simulink model "ElectricVehicle_model_in_the_loop_controller"  (Simulink 8.2)
settings: Solver=ode1  StartTime=0.0  StopTime=42  FixedStep=0.0005  RelTol=1e-3
settings Model: Creator=msdtfa  LastModifiedBy=msdtfa
settings DataIOCC: SignalLoggingName=sigsOut
settings OptimizationCC: ExpressionDepthLimit=128
settings DebuggingCC: SaveWithParameterizedLinksMsg=none  SignalResolutionControl=TryResolveAllWithWarning  SolverPrmCheckMsg=none  MultiTaskDSMMsg=warning  MultiTaskCondExecSysMsg=none  FcnCallInpInsideContextMsg=EnableAllAsError  StateNameClashWarn=none
settings HardwareCC: TargetUnknown=on
settings RTWCC: IncludeERTFirstTime=on

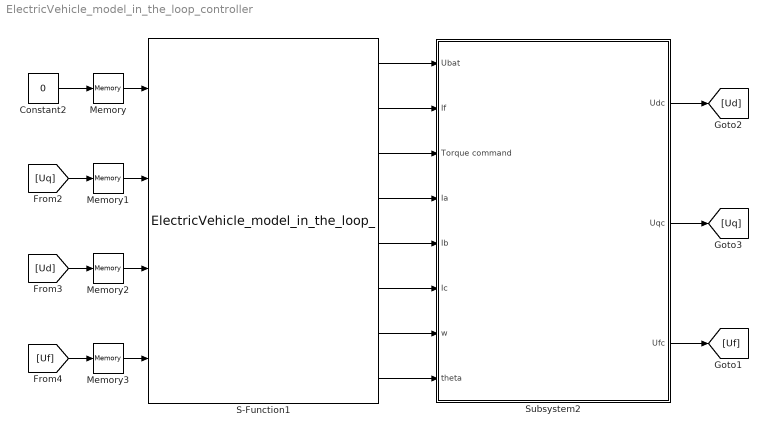
== system ElectricVehicle_model_in_the_loop_controller ==
  Constant2 : Constant  Value=0
  Memory : Memory  InheritSampleTime=on
  Memory1 : Memory  InheritSampleTime=on
  Memory2 : Memory  InheritSampleTime=on
  Memory3 : Memory  X0=500  InheritSampleTime=on
  S-Function1 : S-Function  InitFcn=clear ElectricVehicle_model_in_the_loop_  StopFcn=clear ElectricVehicle_model_in_the_loop_  FunctionName=ElectricVehicle_model_in_the_loop_  Parameters=0.0005 0.01 1e-6  EnableBusSupport=off
      mask Display: port_label('output',1,'Ubat');port_label('output',2,'If');port_label('output',3,'torque_ratio_command');port_label('output',4,'Ia');port_label('output',5,'Ib');port_label('output',6,'Ic');port_label('output',7,'rotary_velocity');port_label('output',8,'mechanical_angle');port_label('input',1,'Uoc');port_label('input',2,'Uqc');port_label('input',3,'Udc');port_label('input',4,'Ufc');disp('Simcenter Amesim:\n ElectricVehicle_model_in_the_loop_')
  Subsystem2 : Subsystem  mask{p=2, Lf=20.8, Rf=35, Tauf=0.01, Msf=0.08, Lsd=0.0006, Lsq=0.0006, Rs=0.08, Taud=0.01, Tauq=0.12, Ifmax=5, Irmsmax=110}
      mask prompts: p "number of pole pairs"; Lf "field winding inductance"; Rf "field winding resistance"; Tauf "field axis PI time constant"; Msf "mutual inductance between stator and field"; Lsd "stator cyclic inductance on Park's d axis"; Lsq "stator cyclic inductance on Park's q axis"; Rs "stator winding resistance"; Taud "d axis PI time constant"; Tauq "q axis PI time constant"; Ifmax "maximum field winding current"; Irmsmax "maximum RMS stator current"
      mask Display:
      | port_label('input',1,'Ubat');
      | port_label('input',2,'If');
      | port_label('input',3,'torque_ratio_c');
      | port_label('input',4,'Ia');
      | port_label('input',5,'Ib');
      | port_label('input',6,'Ic');
      | port_label('input',7,'rotary_velocity');
      | port_label('input',8,'mechanical_angle');
      | port_label('output',1,'Ud');
      | port_label('output',2,'Uq');
      | port_label('output',3,'Uf');
      | 
      | disp('WRSM CONTROL\n Simulink subsystem')
  wires:
  Memory3/1 -> S-Function1/4
  Memory2/1 -> S-Function1/3
  Memory1/1 -> S-Function1/2
  Memory/1 -> S-Function1/1
  Constant2/1 -> Memory/1
  [Uq] -> Memory1/1
  [Uf] -> Memory3/1
  [Ud] -> Memory2/1
  Subsystem2/3(Ufc) -> [Uf]
  Subsystem2/1(Udc) -> [Ud]
  Subsystem2/2(Uqc) -> [Uq]
  S-Function1/3 -> Subsystem2/3(Torque command)
  S-Function1/4 -> Subsystem2/4(Ia)
  S-Function1/5 -> Subsystem2/5(Ib)
  S-Function1/6 -> Subsystem2/6(Ic)
  S-Function1/7 -> Subsystem2/7(w)
  S-Function1/8 -> Subsystem2/8(theta)
  S-Function1/2 -> Subsystem2/2(If)
  S-Function1/1 -> Subsystem2/1(Ubat)

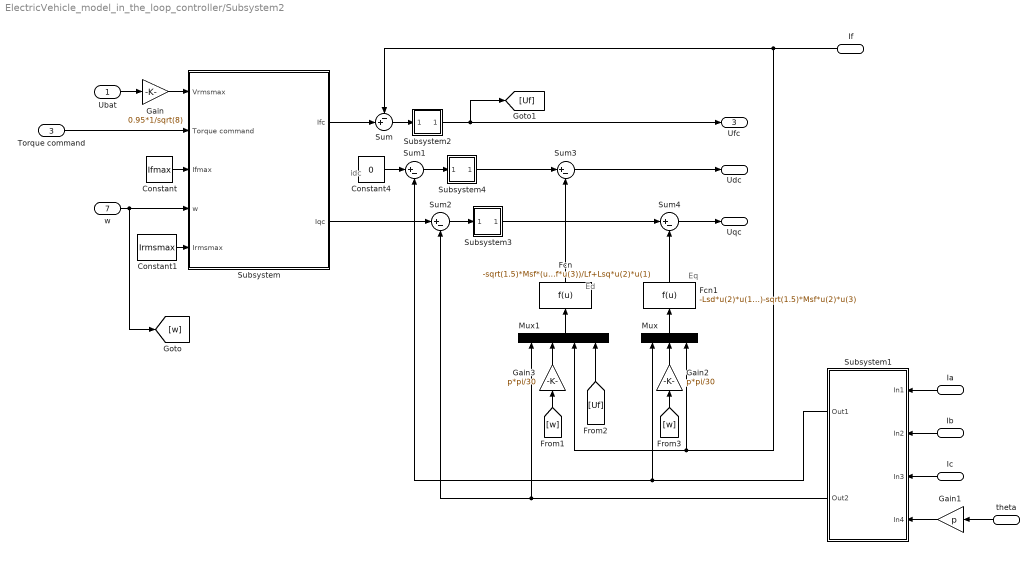
== system ElectricVehicle_model_in_the_loop_controller/Subsystem2 ==
  note: Ed
  note: Eq
  note: idc
  Ubat : Inport
  If : Inport  Port=2
  Torque command : Inport  Port=3
  Ia : Inport  Port=4
  Ib : Inport  Port=5
  Ic : Inport  Port=6
  w : Inport  Port=7
  theta : Inport  Port=8
  Constant : Constant  Value=Ifmax
  Constant1 : Constant  Value=Irmsmax
  Constant4 : Constant  Value=0
  Fcn : Fcn  Expr=-sqrt(1.5)*Msf*(u(4)-Rf*u(3))/Lf+Lsq*u(2)*u(1)
  Fcn1 : Fcn  Expr=-Lsd*u(2)*u(1)-sqrt(1.5)*Msf*u(2)*u(3)
  Gain : Gain  Gain=0.95*1/sqrt(8)  SaturateOnIntegerOverflow=on  OutDataTypeStr=Inherit: Same as input  ParamDataTypeStr=Inherit: Same as input
  Gain1 : Gain  Gain=p  SaturateOnIntegerOverflow=on  OutDataTypeStr=Inherit: Same as input  ParamDataTypeStr=Inherit: Same as input
  Gain2 : Gain  Gain=p*pi/30  SaturateOnIntegerOverflow=on  OutDataTypeStr=Inherit: Same as input  ParamDataTypeStr=Inherit: Same as input
  Gain3 : Gain  Gain=p*pi/30  SaturateOnIntegerOverflow=on  OutDataTypeStr=Inherit: Same as input  ParamDataTypeStr=Inherit: Same as input
  Mux : Mux  Inputs=3
  Mux1 : Mux
  Subsystem : Subsystem  mask{Lsd=Lsd, Lsq=Lsq, Msf=Msf, Rs=Rs, p=p}
      mask prompts: Lsd "stator cyclic inductance on Park's d axis"; Lsq "stator cyclic inductance on Park's q axis"; Msf "mutual inductance between stator and field"; Rs "stator winding resistance"; p "number of pole pairs"
      mask Display:
      | port_label('input',1,'Vrmsmax');
      | port_label('input',2,'Torque_command');
      | port_label('input',3,'Ifmax');
      | port_label('input',4,'rotor_speed');
      | port_label('input',5,'Irmsmax');
      | port_label('output',1,'Ifc');
      | port_label('output',2,'Iqc');
      | disp('WRSM\n torque control')
  Subsystem1 : Subsystem
      mask Display:
      | port_label('input',1,'Ia');
      | port_label('input',2,'Ib');
      | port_label('input',3,'Ic');
      | port_label('input',4,'thetae');
      | 
      | port_label('output',1,'Id');
      | port_label('output',2,'Iq');
      | 
      | disp('abc to dq\ntransformation')
  Subsystem2 : Subsystem  mask{init=500, P=(Lf/Tauf), I=(Rf/Tauf), min=-500, max=500}
      mask prompts: init "initial value"; P "proportional gain"; I "integral gain"; min "minimun value"; max "maximum value"
      mask Display:
      | port_label('output',1,'');
      | port_label('input',1,'');
      | disp('PI sat')
  Subsystem3 : Subsystem  mask{init=0, P=Lsq/Tauq, I=Rs/Tauq, min=-500, max=500}
      mask prompts: init "initial value"; P "proportional gain"; I "integral gain"; min "minimun value"; max "maximum value"
      mask Display:
      | port_label('output',1,'');
      | port_label('input',1,'');
      | disp('PI sat')
  Subsystem4 : Subsystem  mask{init=0, P=(Lsd-3/2*(Msf^2)/Lf)/Taud, I=Rs/Taud, min=-500, max=500}
      mask prompts: init "initial value"; P "proportional gain"; I "integral gain"; min "minimun value"; max "maximum value"
      mask Display:
      | port_label('output',1,'');
      | port_label('input',1,'');
      | disp('PI sat')
  Sum : Sum  Inputs=-+|  SaturateOnIntegerOverflow=on
  Sum{1..4} (4 alike) : Sum  Inputs=|+-  SaturateOnIntegerOverflow=on
  Udc : Outport
  Uqc : Outport  Port=2
  Ufc : Outport  Port=3
  wires:
  Gain/1 -> Subsystem/1(Vrmsmax)
  Constant1/1 -> Subsystem/5(Irmsmax)
  Constant/1 -> Subsystem/3(Ifmax)
  Sum/1 -> Subsystem2/1(In1)
  Gain1/1 -> Subsystem1/4(In4)
  Sum2/1 -> Subsystem3/1(In1)
  Sum1/1 -> Subsystem4/1(In1)
  Constant4/1 -> Sum1/1
  Mux1/1 -> Fcn/1
  Fcn1/1 -> Sum4/2
  Mux/1 -> Fcn1/1
  Sum4/1 -> Uqc/1
  Torque command/1 -> Subsystem/2(Torque command)
  Ia/1 -> Subsystem1/1(In1)
  Ib/1 -> Subsystem1/2(In2)
  Ic/1 -> Subsystem1/3(In3)
  theta/1 -> Gain1/1
  Gain3/1 -> Mux1/2
  Gain2/1 -> Mux/2
  Subsystem2/1(Out1) -> Ufc/1, [Uf]
  Subsystem3/1(Out1) -> Sum4/1
  [w] -> Gain2/1
  If/1 -> Sum/1, Mux/3, Mux1/3
  [Uf] -> Mux1/4
  Ubat/1 -> Gain/1
  Sum3/1 -> Udc/1
  Subsystem4/1(Out1) -> Sum3/1
  Fcn/1 -> Sum3/2
  Subsystem1/2(Out2) -> Mux1/1, Sum2/2
  w/1 -> Subsystem/4(w), [w]
  [w] -> Gain3/1
  Subsystem/1(Ifc) -> Sum/2
  Subsystem/2(Iqc) -> Sum2/1
  Subsystem1/1(Out1) -> Sum1/2, Mux/1

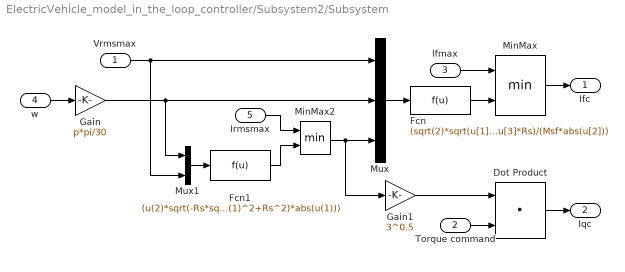
== system ElectricVehicle_model_in_the_loop_controller/Subsystem2/Subsystem ==
  Vrmsmax : Inport
  Torque command : Inport  Port=2
  Ifmax : Inport  Port=3
  w : Inport  Port=4
  Irmsmax : Inport  Port=5
  Dot Product : DotProduct  InputSameDT=on  OutDataTypeStr=Inherit: Inherit via internal rule
  Fcn : Fcn  Expr=(sqrt(2)*sqrt(u[1]^2-u[3]^2*Lsq^2*u[2]^2)-sqrt(2)*u[3]*Rs)/(Msf*abs(u[2]))
  Fcn1 : Fcn  Expr=(u(2)*sqrt(-Rs*sqrt(Lsq^2*u(1)^2+Rs^2)+Lsq^2*u(1)^2+Rs^2))/(sqrt(2)*Lsq*sqrt(Lsq^2*u(1)^2+Rs^2)*abs(u(1)))
  Gain : Gain  Gain=p*pi/30  SaturateOnIntegerOverflow=on  OutDataTypeStr=Inherit: Same as input  ParamDataTypeStr=Inherit: Same as input
  Gain1 : Gain  Gain=3^0.5  SaturateOnIntegerOverflow=on  OutDataTypeStr=Inherit: Same as input  ParamDataTypeStr=Inherit: Same as input
  MinMax : MinMax  Inputs=2  SaturateOnIntegerOverflow=on  InputSameDT=on
  MinMax2 : MinMax  Inputs=2  SaturateOnIntegerOverflow=on  InputSameDT=on
  Mux : Mux  Inputs=3
  Mux1 : Mux  Inputs=2
  Ifc : Outport
  Iqc : Outport  Port=2
  wires:
  Vrmsmax/1 -> Mux/1, Mux1/2
  Gain/1 -> Mux1/1, Mux/2
  Fcn/1 -> MinMax/2
  Mux1/1 -> Fcn1/1
  MinMax2/1 -> Mux/3, Gain1/1
  Fcn1/1 -> MinMax2/2
  Mux/1 -> Fcn/1
  Dot Product/1 -> Iqc/1
  Ifmax/1 -> MinMax/1
  MinMax/1 -> Ifc/1
  w/1 -> Gain/1
  Irmsmax/1 -> MinMax2/1
  Gain1/1 -> Dot Product/1
  Torque command/1 -> Dot Product/2

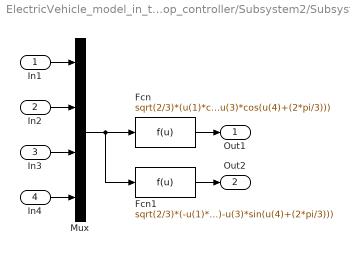
== system ElectricVehicle_model_in_the_loop_controller/Subsystem2/Subsystem1 ==
  In1 : Inport
  In2 : Inport  Port=2
  In3 : Inport  Port=3
  In4 : Inport  Port=4
  Fcn : Fcn  Expr=sqrt(2/3)*(u(1)*cos(u(4))+u(2)*cos(u(4)-(2*pi/3))+u(3)*cos(u(4)+(2*pi/3)))
  Fcn1 : Fcn  Expr=sqrt(2/3)*(-u(1)*sin(u(4))-u(2)*sin(u(4)-(2*pi/3))-u(3)*sin(u(4)+(2*pi/3)))
  Mux : Mux
  Out1 : Outport
  Out2 : Outport  Port=2
  wires:
  Mux/1 -> Fcn/1, Fcn1/1
  In1/1 -> Mux/1
  In2/1 -> Mux/2
  In3/1 -> Mux/3
  Fcn/1 -> Out1/1
  In4/1 -> Mux/4
  Fcn1/1 -> Out2/1

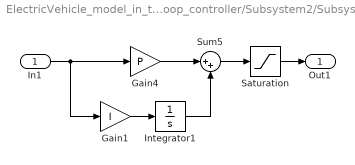
== system ElectricVehicle_model_in_the_loop_controller/Subsystem2/Subsystem2 ==
  In1 : Inport
  Gain1 : Gain  Gain=I  SaturateOnIntegerOverflow=on  OutDataTypeStr=Inherit: Same as input  ParamDataTypeStr=Inherit: Same as input
  Gain4 : Gain  Gain=P  SaturateOnIntegerOverflow=on  OutDataTypeStr=Inherit: Same as input  ParamDataTypeStr=Inherit: Same as input
  Integrator1 : Integrator  InitialCondition=init  LimitOutput=on  UpperSaturationLimit=max  LowerSaturationLimit=min
  Saturation : Saturate  UpperLimit=max  LowerLimit=min
  Sum5 : Sum  Inputs=|++  SaturateOnIntegerOverflow=on
  Out1 : Outport
  wires:
  Gain4/1 -> Sum5/1
  Integrator1/1 -> Sum5/2
  In1/1 -> Gain4/1, Gain1/1
  Sum5/1 -> Saturation/1
  Saturation/1 -> Out1/1
  Gain1/1 -> Integrator1/1

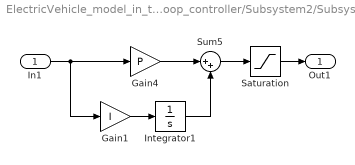
== system ElectricVehicle_model_in_the_loop_controller/Subsystem2/Subsystem3 ==
  In1 : Inport
  Gain1 : Gain  Gain=I  SaturateOnIntegerOverflow=on  OutDataTypeStr=Inherit: Same as input  ParamDataTypeStr=Inherit: Same as input
  Gain4 : Gain  Gain=P  SaturateOnIntegerOverflow=on  OutDataTypeStr=Inherit: Same as input  ParamDataTypeStr=Inherit: Same as input
  Integrator1 : Integrator  InitialCondition=init  LimitOutput=on  UpperSaturationLimit=max  LowerSaturationLimit=min
  Saturation : Saturate  UpperLimit=max  LowerLimit=min
  Sum5 : Sum  Inputs=|++  SaturateOnIntegerOverflow=on
  Out1 : Outport
  wires:
  Gain4/1 -> Sum5/1
  Integrator1/1 -> Sum5/2
  In1/1 -> Gain4/1, Gain1/1
  Sum5/1 -> Saturation/1
  Saturation/1 -> Out1/1
  Gain1/1 -> Integrator1/1

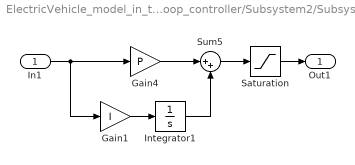
== system ElectricVehicle_model_in_the_loop_controller/Subsystem2/Subsystem4 ==
  In1 : Inport
  Gain1 : Gain  Gain=I  SaturateOnIntegerOverflow=on  OutDataTypeStr=Inherit: Same as input  ParamDataTypeStr=Inherit: Same as input
  Gain4 : Gain  Gain=P  SaturateOnIntegerOverflow=on  OutDataTypeStr=Inherit: Same as input  ParamDataTypeStr=Inherit: Same as input
  Integrator1 : Integrator  InitialCondition=init  LimitOutput=on  UpperSaturationLimit=max  LowerSaturationLimit=min
  Saturation : Saturate  UpperLimit=max  LowerLimit=min
  Sum5 : Sum  Inputs=|++  SaturateOnIntegerOverflow=on
  Out1 : Outport
  wires:
  Gain4/1 -> Sum5/1
  Integrator1/1 -> Sum5/2
  In1/1 -> Gain4/1, Gain1/1
  Sum5/1 -> Saturation/1
  Saturation/1 -> Out1/1
  Gain1/1 -> Integrator1/1
